simulink model "SIMULACAO_PROJETO_3_0"  (R2022a)
settings: Solver=VariableStepAuto  StartTime=0.0  StopTime=5500  RelTol=1e-3
libraries: cstblocks x6
settings Model: Creator=allti  LastModifiedBy=allti

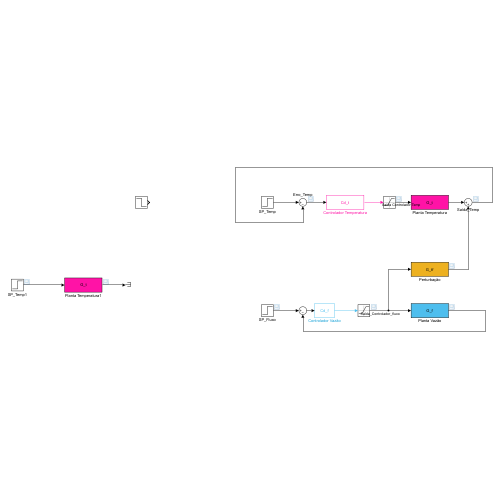
[thumbnail: Simulink's stored preview of the top-level diagram]
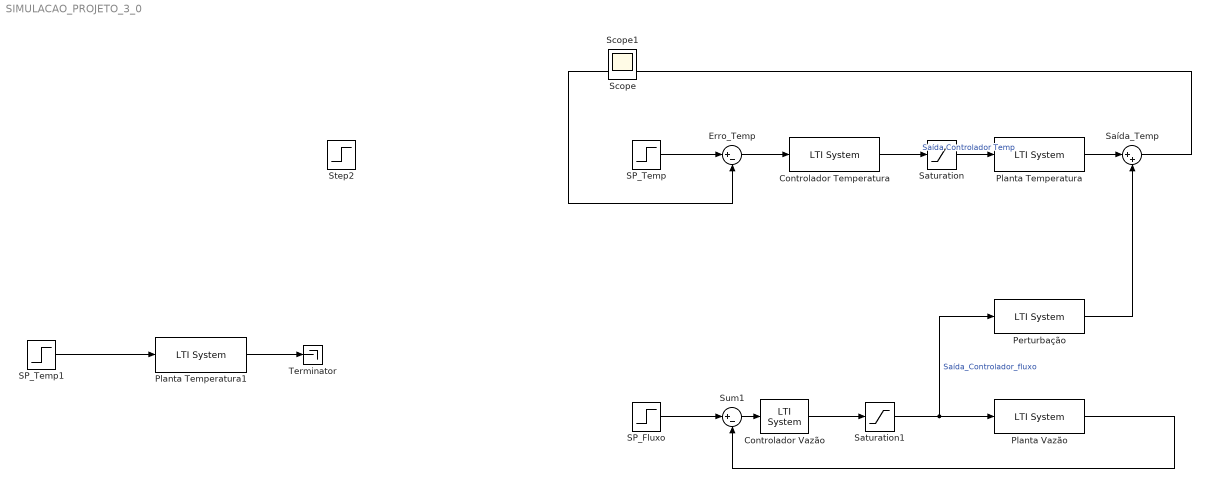
== system SIMULACAO_PROJETO_3_0 ==
  Controlador Temperatura : cstblocks/LTI System  sys=Cd_t  IC=[]
  Controlador Vazão : cstblocks/LTI System  sys=Cd_f  IC=[]
  Erro_Temp : Sum  Inputs=|+-
  Perturbação : cstblocks/LTI System  sys=G_tf  IC=[]
  Planta Temperatura : cstblocks/LTI System  sys=G_t  IC=[]
  Planta Temperatura1 : cstblocks/LTI System  sys=G_t  IC=[]
  Planta Vazão : cstblocks/LTI System  sys=G_f  IC=[]
  SP_Fluxo : Step  Time=2000  After=8  SampleTime=0
  SP_Temp : Step  Time=0  After=46.05-26.05  SampleTime=0
  SP_Temp1 : Step  Time=0  After=61.17  SampleTime=0
  Saturation : Saturate  UpperLimit=255  LowerLimit=0
  Saturation1 : Saturate  UpperLimit=255  LowerLimit=0
  Saída_Temp : Sum  Inputs=|++
  Step2 : Step  Time=4100  After=-5  SampleTime=0
  Sum1 : Sum  Inputs=|+-
  Terminator : Terminator
  Scope : Scope
  Scope1 : Scope
  wires:
  Erro_Temp/1 -> Controlador Temperatura/1
  SP_Fluxo/1 -> Sum1/1
  Sum1/1 -> Controlador Vazão/1
  Planta Vazão/1 -> Sum1/2
  Planta Temperatura/1 -> Saída_Temp/1
  Saída_Temp/1 -> Erro_Temp/2
  Perturbação/1 -> Saída_Temp/2
  SP_Temp/1 -> Erro_Temp/1
  Controlador Temperatura/1 -> Saturation/1
  Saturation/1 -> Planta Temperatura/1  "Saída Controlador Temp"
  Controlador Vazão/1 -> Saturation1/1
  Saturation1/1 -> Perturbação/1, Planta Vazão/1  "Saída_Controlador_fluxo"
  SP_Temp1/1 -> Planta Temperatura1/1
  Planta Temperatura1/1 -> Terminator/1
